simulink model "MotorXploer (1)"  (R2025a)
settings: Solver=FixedStepAuto  StartTime=0.0  StopTime=inf  FixedStep=0.001  RelTol=1e-3
undefined symbols (not defined in the file): Blocking, LF, Non
libraries: amg_usbconverter_n_connect_lib x3, eeGeneralControl x3, dspstat3 x1
settings Model: Creator=beamk  LastModifiedBy=User

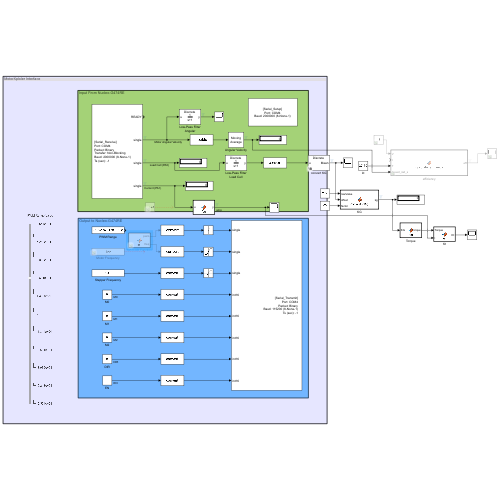
[thumbnail: Simulink's stored preview of the top-level diagram]
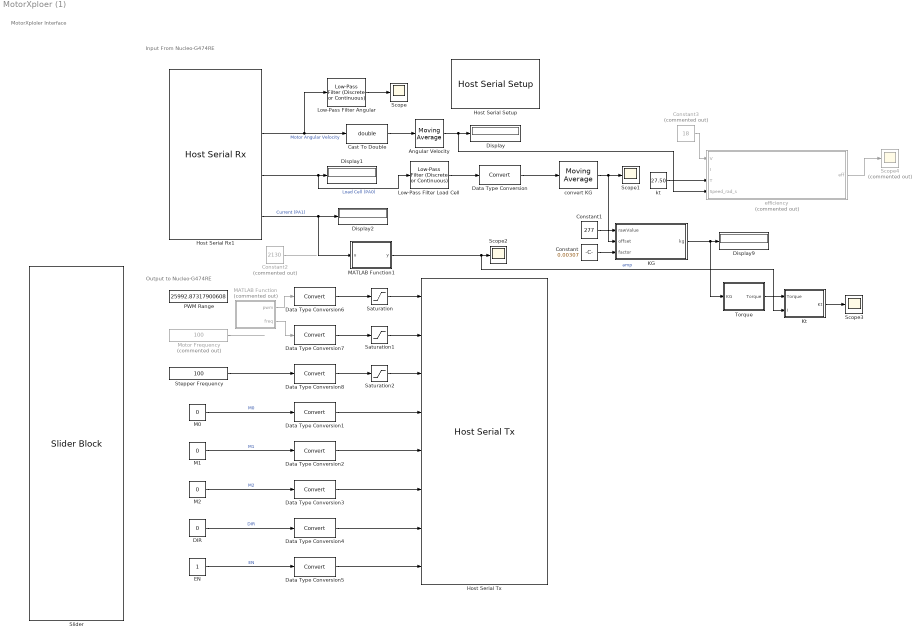
== system MotorXploer (1) ==
  note: Output to Nucleo-G474RE
  note: Input From Nucleo-G474RE
  note: MotorXploler Interface
  Angular Velocity : dspstat3/Moving Average  Method=Sliding window  ForgettingFactorPort=off  SpecifyWindowLength=on  WindowLength=4  OverlapLength=3  AllowArbitraryInputLength=off  ForgettingFactor=0.9  SimulateUsing=Interpreted execution
  Cast To Double : DataTypeConversion  OutDataTypeStr=double  SaturateOnIntegerOverflow=off  RndMeth=Floor
  Constant : Constant  Value=0.00307
  Constant1 : Constant  Value=277
  Constant2 : Constant  Commented=on  Value=2130
  Constant3 : Constant  Commented=on  Value=18
  DIR : Constant  Value=0
  Data Type Conversion{,1..8} (9 alike) : DataTypeConversion  SaturateOnIntegerOverflow=off  RndMeth=Floor
  Display{,1..2,9} (4 alike) : Display
  EN : Constant
  Host Serial Rx1 : amg_usbconverter_n_connect_lib/Host Serial Rx  conf=rx  port=COM4  baudrate=2000000  databits=8  parity=None  stopbit=1  flowcontrol=None  transfer=Non-Blocking  timeout=5  packetmode=Binary  enableinitialvalues=off  initialvalues=[]  binheader='25'  binterminator='4E'  porttype_double=0  porttype_single=3  porttype_int8=0  porttype_uint8=0  porttype_int16=0  porttype_uint16=0  porttype_int32=0  porttype_uint32=0  asciiformat='%f,%f,%d,%d'  rx_asciiterminator="LF (0x0A - \"\\n\")"  tx_asciiterminator="CRLF (0x0D 0x0A - \"\\r\\n\")"  sampletime=-1  enablecustomportlabel=off  cinputportlabel=0  coutputportlabel=A  portpinstr=0  blockid=HostSerialRx1  inputporttype=[]  inputportwidth=[]  inputportlabel={}  outputporttype=[3 1 1 1]  outputportwidth=[1 1 1 1]  outputportlabel={'READY','single','single','single'}  compat=0  optionstring=[]  autoport='COM4'
  Host Serial Setup : amg_usbconverter_n_connect_lib/Host Serial Setup  conf=setup  port=COM4  baudrate=2000000  databits=8  parity=None  stopbit=1  flowcontrol=None  transfer=Blocking  timeout=2  packetmode=Binary  initialvalues=[]  binheader='7E 7E'  binterminator='03 03'  porttype_double=0  porttype_single=1  porttype_int8=0  porttype_uint8=0  porttype_int16=0  porttype_uint16=0  porttype_int32=0  porttype_uint32=2  asciiformat='%d %u %x'  rx_asciiterminator="CRLF (0x0D 0x0A - \"\\r\\n\")"  tx_asciiterminator="CRLF (0x0D 0x0A - \"\\r\\n\")"  sampletime=-1  enablecustomportlabel=off  cinputportlabel=0  coutputportlabel=A  portpinstr=0  blockid=HostSerialSetup  inputporttype=[]  inputportwidth=[]  inputportlabel={}  outputporttype=[]  outputportwidth=[]  outputportlabel={}  compat=0  optionstring=[]  autoport='COM4'
  Host Serial Tx : amg_usbconverter_n_connect_lib/Host Serial Tx  conf=tx  port=<auto>  baudrate=115200  databits=8  parity=None  stopbit=1  flowcontrol=None  transfer=Blocking  timeout=2  packetmode=Binary  initialvalues=[]  binheader='25'  binterminator='4E'  porttype_double=0  porttype_single=3  porttype_int8=0  porttype_uint8=0  porttype_int16=5  porttype_uint16=0  porttype_int32=0  porttype_uint32=0  asciiformat='%d,%f'  rx_asciiterminator="CRLF (0x0D 0x0A - \"\\r\\n\")"  tx_asciiterminator="CRLF (0x0D 0x0A - \"\\r\\n\")"  sampletime=-1  enablecustomportlabel=off  cinputportlabel=0  coutputportlabel=A  portpinstr=0  blockid=HostSerialTx  inputporttype=[1 1 1 4 4 4 4 4]  inputportwidth=[1 1 1 1 1 1 1 1]  inputportlabel={'single','single','single','int16','int16','int16','int16','int16'}  outputporttype=[]  outputportwidth=[]  outputportlabel={}  compat=0  optionstring=[]  autoport='COM4'
      settings: SourceProductName=aMG USB Converter N
  KG : MATLAB Function  TreatAsAtomicUnit=on
  Kt : MATLAB Function  TreatAsAtomicUnit=on
  Low-Pass Filter Angular : eeGeneralControl/Low-Pass Filter (Discrete or Continuous)  K=1  T=1  B=inf  A=-inf  init_option=Inherited from block input  x0=0  Ts=-1
  Low-Pass Filter Load Cell : eeGeneralControl/Low-Pass Filter (Discrete or Continuous)  K=1  T=1  B=inf  A=-inf  init_option=Inherited from block input  x0=0  Ts=-1
  M0 : Constant  Value=0
  M1 : Constant  Value=0
  M2 : Constant  Value=0
  MATLAB Function : MATLAB Function  Commented=on  TreatAsAtomicUnit=on
  MATLAB Function1 : MATLAB Function  TreatAsAtomicUnit=on
  Motor Frequency : Constant  Commented=on  Value=100  OutDataTypeStr=single
  PWM Range : Constant  Value=25992.87317900608  OutDataTypeStr=single
  Saturation : Saturate  UpperLimit=65535  LowerLimit=-65535
  Saturation1 : Saturate  UpperLimit=20000  LowerLimit=0
  Saturation2 : Saturate  UpperLimit=inf  LowerLimit=0
  Scope{,1..3} (4 alike) : Scope
      Scope settings: ActiveDisplayYMinimum=-18.947306432810066  ActiveDisplayYMaximum=160.57332562263713
      Scope1 settings: ActiveDisplayYMinimum=-71.560299650587439  ActiveDisplayYMaximum=412.34669028244855
      Scope2 settings: ActiveDisplayYMinimum=-0.341703286576271  ActiveDisplayYMaximum=1.8023295791864395  DataLoggingVariableName=ScopeData2
      Scope3 settings: DataLoggingVariableName=ScopeData3
  Scope4 : Scope  Commented=on
      settings: DataLoggingVariableName=ScopeData4
  Slider : SliderBlock  ScaleMin=-65535  ScaleMax=65535
  Stepper Frequency : Constant  Value=100  OutDataTypeStr=single
  Torque : MATLAB Function  TreatAsAtomicUnit=on
  convert KG : eeGeneralControl/Moving Average  VariantControl=Variant1  LabelModeActiveChoice=Discrete  f=60  x0=0  BufferSize=8192  Ts=-1
      settings: LibrarySourceBlock=ee_sl_lib/General Control/Moving Average
  efficiency : MATLAB Function  Commented=on  TreatAsAtomicUnit=on
  kt : Constant  Value=27.50
  wires:
  Host Serial Rx1/2 -> Low-Pass Filter Angular/1, Cast To Double/1  "Motor Angular Velocity"
  Host Serial Rx1/3 -> Low-Pass Filter Load Cell/1, Display1/1  "Load Cell (PA0)"
  M0/1 -> Data Type Conversion1/1  "M0"
  EN/1 -> Data Type Conversion5/1  "EN"
  DIR/1 -> Data Type Conversion4/1  "DIR"
  M1/1 -> Data Type Conversion2/1  "M1"
  M2/1 -> Data Type Conversion3/1  "M2"
  Motor Frequency/1 -> ?
  Stepper Frequency/1 -> Data Type Conversion8/1
  Data Type Conversion1/1 -> Host Serial Tx/4
  Data Type Conversion2/1 -> Host Serial Tx/5
  Data Type Conversion3/1 -> Host Serial Tx/6
  Data Type Conversion4/1 -> Host Serial Tx/7
  Data Type Conversion5/1 -> Host Serial Tx/8
  Data Type Conversion6/1 -> Saturation/1
  Saturation/1 -> Host Serial Tx/1
  Data Type Conversion7/1 -> Saturation1/1
  Data Type Conversion8/1 -> Saturation2/1
  MATLAB Function/1(pwm) -> Data Type Conversion6/1
  Saturation1/1 -> Host Serial Tx/2
  Saturation2/1 -> Host Serial Tx/3
  Host Serial Rx1/4 -> MATLAB Function1/1(u), Display2/1  "Current (PA1)"
  KG/1(kg) -> Torque/1(KG), Display9/1
  convert KG/1 -> KG/1(rawValue), Scope1/1
  Data Type Conversion/1 -> convert KG/1
  Constant1/1 -> KG/2(offset)
  Constant/1 -> KG/3(factor)
  Low-Pass Filter Angular/1 -> Scope/1
  Constant2/1 -> ?
  MATLAB Function/2(freq) -> Data Type Conversion7/1
  Angular Velocity/1 -> efficiency/4(Speed_rad_s), Display/1
  Cast To Double/1 -> Angular Velocity/1
  Low-Pass Filter Load Cell/1 -> Data Type Conversion/1
  MATLAB Function1/1(y) -> Kt/2(I), Scope2/1  "amp"
  Torque/1(Torque) -> Kt/1(Torque)
  Kt/1(Kt) -> Scope3/1
  Constant3/1 -> efficiency/1(V)
  efficiency/1(eff) -> Scope4/1
  kt/1 -> efficiency/3(T)

== matlab function MotorXploer (1)/Kt ==
  data: Torque input; Kt output; I input
function Kt = fcn(Torque,I)

Kt = Torque/I;

== matlab function MotorXploer (1)/Torque ==
  data: KG input; Torque output
function Torque = fcn(KG)

Torque = KG * 9.81 * 110.5;

== matlab function MotorXploer (1)/efficiency ==
  data: V input; eff output; I input; T input; Speed_rad_s input
function eff  = calculate_efficiency(V, I, T, Speed_rad_s)
    % calculate_efficiency คำนวณค่าประสิทธิภาพมอเตอร์
    % Inputs:
    %   V           : แรงดันไฟฟ้า (Volts) -> 24V
    %   I           : กระแสไฟฟ้า (Amps) -> จาก WCS1600
    %   T           : แรงบิด (N.m) -> จาก Load Cell
    %   Speed_rad_s : ความเร็วเชิงมุม (rad/s) -> จาก Encoder
    % Outputs:
    %   eff   : ประสิทธิภาพ (%)
    %   P_in  : กำลังไฟฟ้าขาเข้า (Watts)
    %   P_out : กำลังกลขาออก (Watts)

    % 1. คำนวณกำลังไฟฟ้าขาเข้า (Electrical Power Input)
    % สูตร: P = V * I
    P_in = V * I;

    % 2. คำนวณกำลังกลขาออก (Mechanical Power Output)
    % สูตร: P = Torque * Omega
    P_out = T * Speed_rad_s;

    % 3. คำนวณประสิทธิภาพ (Efficiency)
    % สูตร: eta = (P_out / P_in) * 100
   
end

== matlab function MotorXploer (1)/KG ==
  data: rawValue input; kg output; offset input; factor input
function kg = convertToKg(rawValue, offset, factor)
% This function converts a raw ADC value to kilograms
%
% Inputs:
%   rawValue = ค่าดิบที่อ่านได้จากเซ็นเซอร์
%   offset   = ค่าดิบที่อ่านได้ตอนน้ำหนักเป็น 0 (ค่า Tare)
%   factor   = ค่าตัวคูณสำหรับแปลงค่า (ที่คำนวณไว้)

% คำนวณน้ำหนัก
weight = (rawValue - offset) * factor;

% (ทางเลือก) ป้องกันน้ำหนักติดลบ หากค่าสั่นไหว
if weight < 0
    kg = 0;
else
    kg = weight;
end

end

== matlab function MotorXploer (1)/MATLAB Function ==
  data: pwm output; freq output
function [pwm, freq] = fcn()

persistent freqList pwmStep sampleCount freqIndex pwmIndex roundCount;

% Initialize
if isempty(freqList)
    freqList = [80000 80000 80000];
    pwmStep = 0:0.05:1.0; 
    %pwmStep = 0:0.1:1.0; 
    sampleCount = 0;
    freqIndex = 1;
    pwmIndex = 1;
    roundCount = 1;
end

% Stop after 4 rounds
if roundCount > 1
    pwm = 0;
    freq = 0;
    return;
end

% Output 
freq = freqList(freqIndex);
pwm  = pwmStep(pwmIndex) * (65535);   % <-- ตอนนี้เป็น double แล้ว

% Update counter
sampleCount = sampleCount + 1;

if sampleCount >= 10000
    sampleCount = 0;
    pwmIndex = pwmIndex + 1;

    if pwmIndex > length(pwmStep)
        pwmIndex = 1;
        freqIndex = freqIndex + 1;

        if freqIndex > length(freqList)
            freqIndex = 1;
            roundCount = roundCount + 1;
        end
    end
end

== matlab function MotorXploer (1)/MATLAB Function1 ==
  data: u input; y output
function y = fcn(u)

y = (u - 2112.2) * 1/29.469;
